simulink model "Wheelsimmod"  (R2023a)
settings: Solver=VariableStepAuto  StartTime=0.0  StopTime=4  RelTol=1e-3
values from neighbouring files (symbols this model uses):
  mass = 1    [rovervars.mat]    (also in varedit.m)
  radius = 0.1    [rovervars.mat]    (also in varedit.m)
  stepTime = 2    [rovervars.mat]    (also in varedit.m)
  torqueF = 0.05    [rovervars.mat]    (also in varedit.m)
settings Model: Creator=MY DELL  LastModifiedBy=MY DELL

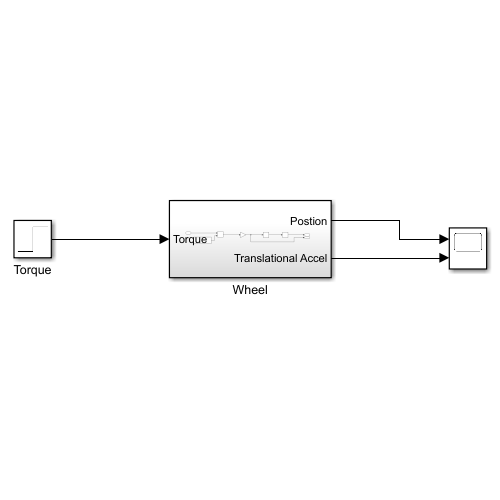
[thumbnail: Simulink's stored preview of the top-level diagram]
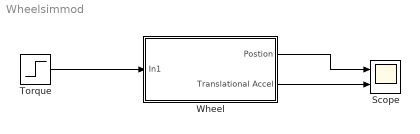
== system Wheelsimmod ==
  Scope : Scope  NumInputPorts=2
  Torque : Step  Time=stepTime  After=torqueF  SampleTime=0
  Wheel : Subsystem
  wires:
  Torque/1 -> Wheel/1(In1)
  Wheel/1(Postion) -> Scope/1
  Wheel/2(Translational Accel) -> Scope/2

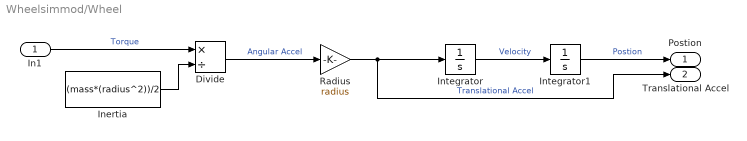
== system Wheelsimmod/Wheel ==
  In1 : Inport
  Divide : Product  Inputs=*/
  Inertia : Constant  Value=(mass*(radius^2))/2
  Integrator : Integrator
  Integrator1 : Integrator
  Radius : Gain  Gain=radius
  Postion : Outport
  Translational Accel : Outport  Port=2
  wires:
  Integrator/1 -> Integrator1/1  "Velocity"
  Inertia/1 -> Divide/2
  Divide/1 -> Radius/1  "Angular Accel"
  Radius/1 -> Translational Accel/1, Integrator/1  "Translational Accel"
  Integrator1/1 -> Postion/1  "Postion"
  In1/1 -> Divide/1  "Torque"
